simulink model "sf_truthtable"  (R2015b)
settings: Solver=ode45  StartTime=0.0  StopTime=1  RelTol=1e-3
settings Model: Creator=amatsumo  LastModifiedBy=amatsumo
settings DataIOCC: SaveFormat=Array
settings DebuggingCC: UnderspecifiedInitializationDetection=Classic  MergeDetectMultiDrivingBlocksExec=none  SolverPrmCheckMsg=warning  StateNameClashWarn=warning
settings HardwareCC: ProdBitPerPointer=32  ProdLargestAtomicFloat=None  ProdIntDivRoundTo=Undefined  ProdEndianess=Unspecified  ProdWordSize=32  ProdHWDeviceType=32-bit Generic
settings GRTTargetCC: GeneratePreprocessorConditionals=Disable all
settings ConfigComp: CovModelRefEnable=Off  CovSFcnEnable=off

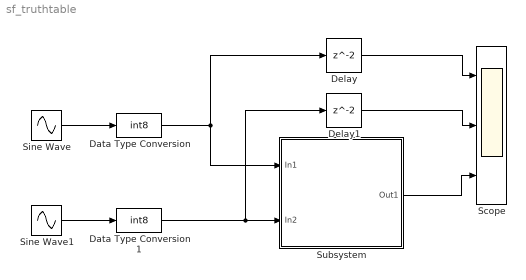
== system sf_truthtable ==
  Data Type Conversion : DataTypeConversion  OutDataTypeStr=int8
  Data Type Conversion1 : DataTypeConversion  OutDataTypeStr=int8
  Delay : Delay
  Delay1 : Delay
  Scope : Scope  NumInputPorts=3
  Sine Wave : Sin  Amplitude=127  Frequency=2*pi*5  SampleTime=1/100
  Sine Wave1 : Sin  Amplitude=127  Frequency=2*pi*8  SampleTime=1/100
  Subsystem : Subsystem
  wires:
  Sine Wave/1 -> Data Type Conversion/1
  Sine Wave1/1 -> Data Type Conversion1/1
  Delay1/1 -> Scope/2
  Delay/1 -> Scope/1
  Subsystem/1(Out1) -> Scope/3
  Data Type Conversion/1 -> Delay/1, Subsystem/1(In1)
  Data Type Conversion1/1 -> Delay1/1, Subsystem/2(In2)

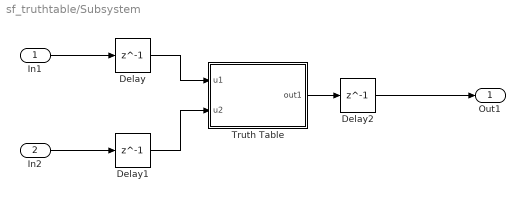
== system sf_truthtable/Subsystem ==
  In1 : Inport
  In2 : Inport  Port=2
  Delay : Delay  DelayLength=1
  Delay1 : Delay  DelayLength=1
  Delay2 : Delay  DelayLength=1
  Truth Table : Truth Table  TreatAsAtomicUnit=on
  Out1 : Outport
  wires:
  Delay2/1 -> Out1/1
  Delay1/1 -> Truth Table/2(u2)
  In2/1 -> Delay1/1
  Delay/1 -> Truth Table/1(u1)
  Truth Table/1(out1) -> Delay2/1
  In1/1 -> Delay/1

== matlab function sf_truthtable/Subsystem/Truth Table ==
  data: u1 input int8; out1 output uint8; u2 input int8
function out1 = fcn(u1, u2)

aVarTruthTableCondition_1 = false;
aVarTruthTableCondition_2 = false;


% Example condition 1

aVarTruthTableCondition_1 = logical(u1 >= 0);

% Example condition 2

aVarTruthTableCondition_2 = logical(u2 >= 0);

if (aVarTruthTableCondition_1 && ~aVarTruthTableCondition_2)
    Action1();
elseif (~aVarTruthTableCondition_1 && aVarTruthTableCondition_2)
    Action2();
elseif (aVarTruthTableCondition_1 && aVarTruthTableCondition_2)
    Action3();
else % Default
    Action4();
end

function Action1()


out1 = uint8(1);

function Action2()


out1 = uint8(2);

function Action3()


out1 = uint8(3);

function Action4()


out1 = uint8(4);
